simulink model "DC_motor_MRAC_c"  (R2016a)
settings: Solver=VariableStepAuto  StartTime=0.0  StopTime=20  MaxStep=0.01  RelTol=1e-3
undefined symbols (not defined in the file): Am, Bm, Cm, Gammae, Gammau, Gammax
settings Model: Creator=mgreiff  LastModifiedBy=mgreiff
settings DataIOCC: LimitDataPoints=on
settings DebuggingCC: AllowSymbolicDim=off
settings ModelReferenceCC: PropagateSignalLabelsOutOfModel=off
settings GRTTargetCC: GeneratePreprocessorConditionals=Use local settings

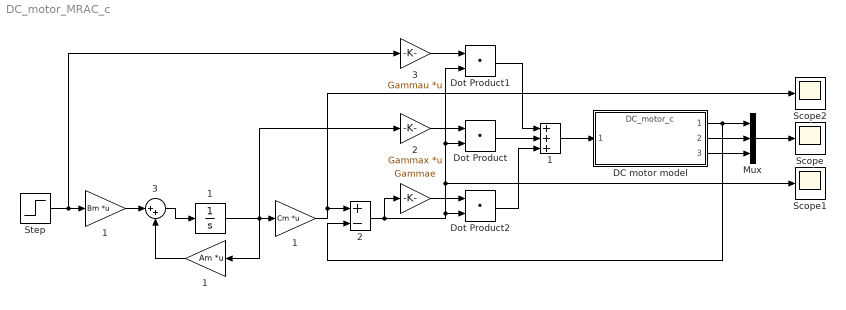
== system DC_motor_MRAC_c ==
  "   " : Gain  Gain=Gammae
  "       1" : Gain  Gain=Cm  Multiplication=Matrix(K*u)
  "    1" : Gain  Gain=Am  Multiplication=Matrix(K*u)
  "    2" : Gain  Gain=Gammax  Multiplication=Matrix(K*u)
  "    3" : Gain  Gain=Gammau  Multiplication=Matrix(K*u)
  "   1" : Integrator
  "  1" : Gain  Gain=Bm  Multiplication=Matrix(K*u)
  " 1" : Sum  Inputs=+++
  " 2" : Sum  Inputs=+-
  " 3" : Sum  Inputs=|++
  DC motor model : ModelReference  ModelNameDialog=DC_motor_c.slx  SimulationMode=Normal  ModelReferenceVersion=1.8
  Dot Product : DotProduct  InputSameDT=on  OutDataTypeStr=Inherit: Inherit via internal rule
  Dot Product1 : DotProduct  InputSameDT=on  OutDataTypeStr=Inherit: Inherit via internal rule
  Dot Product2 : DotProduct  InputSameDT=on  OutDataTypeStr=Inherit: Inherit via internal rule
  Mux : Mux  Inputs=3
  Scope : Scope
  Scope1 : Scope
  Scope2 : Scope
  Step : Step  Time=0  After=2  SampleTime=0
  wires:
  " 3"/1 -> "   1"/1
  "  1"/1 -> " 3"/1
  "    1"/1 -> " 3"/2
  "   1"/1 -> "    2"/1, "    1"/1, "       1"/1
  "       1"/1 -> Scope2/1, " 2"/1
  " 2"/1 -> Dot Product2/2, Dot Product1/2, Dot Product/2, Scope1/1, "   "/1
  Step/1 -> "    3"/1, "  1"/1
  Dot Product/1 -> " 1"/2
  Dot Product1/1 -> " 1"/1
  " 1"/1 -> DC motor model/1
  "    2"/1 -> Dot Product/1
  "    3"/1 -> Dot Product1/1
  Dot Product2/1 -> " 1"/3
  "   "/1 -> Dot Product2/1
  DC motor model/3 -> Mux/3
  DC motor model/1 -> " 2"/2, Mux/1
  DC motor model/2 -> Mux/2
  Mux/1 -> Scope/1
